simulink model "ex1"  (R2020a)
settings: Solver=VariableStepAuto  StartTime=0.0  StopTime=10.0  RelTol=1e-3

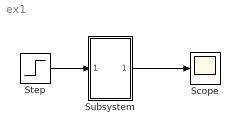
== system ex1 ==
  Scope : Scope
  Step : Step  SampleTime=0
  Subsystem : Subsystem  mask{a=12}
      mask prompts: a "a="
      mask init:
      | if str2num(get_param(gcb,'a'))<0
      | error('Introduceti o variabila pozitiva!')
      | end
  wires:
  Step/1 -> Subsystem/1(In1)
  Subsystem/1(Out1) -> Scope/1

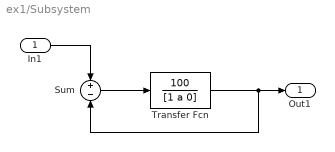
== system ex1/Subsystem ==
  In1 : Inport
  Sum : Sum  Inputs=+-
  Transfer Fcn : TransferFcn  Numerator=[100]  Denominator=[1 a 0]
  Out1 : Outport
  wires:
  Sum/1 -> Transfer Fcn/1
  In1/1 -> Sum/1
  Transfer Fcn/1 -> Out1/1, Sum/2
